simulink subsystem "Szakaszmotornelkul"  (R2024b)
settings: Solver=VariableStepAuto  StartTime=0.0  StopTime=10.0  RelTol=1e-3
undefined symbols (not defined in the file or in its folder): tau_max
settings Model: Creator=Asus  LastModifiedBy=Asus

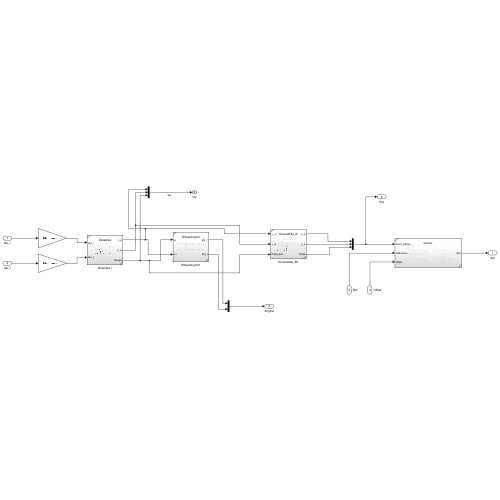
[thumbnail: Simulink's stored preview of the top-level diagram]
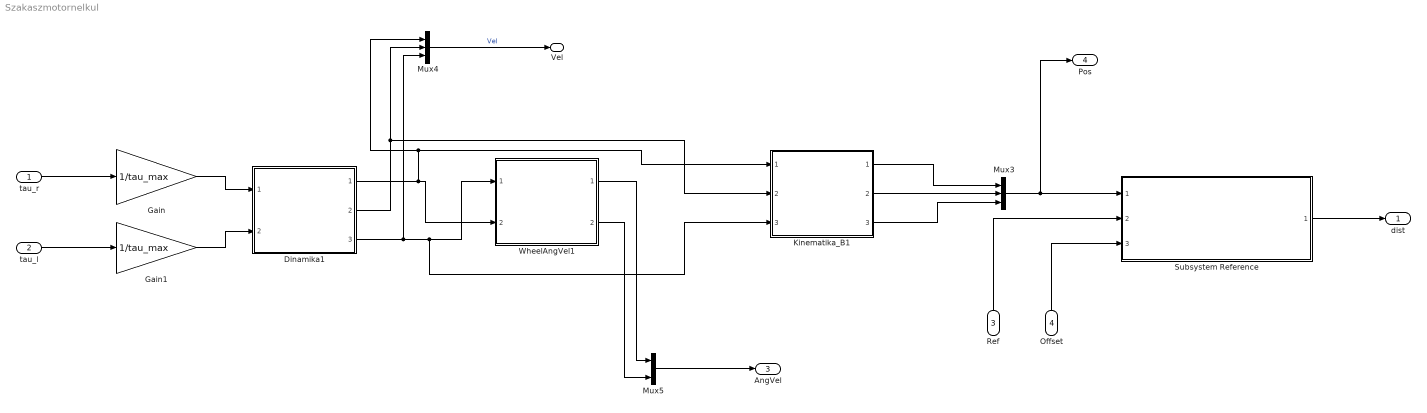
== system Szakaszmotornelkul ==
  tau_r : Inport
  tau_l : Inport  Port=2
  Ref : Inport  Port=3
  Offset : Inport  Port=4
  Dinamika1 : Subsystem  ReferencedSubsystem=Dinamika
  Gain : Gain  Gain=1/tau_max
  Gain1 : Gain  Gain=1/tau_max
  Kinematika_B1 : Subsystem  ReferencedSubsystem=Kinematika_B
  Mux3 : Mux  Inputs=3
  Mux4 : Mux  Inputs=3
  Mux5 : Mux  Inputs=2
  Subsystem Reference : Subsystem  ReferencedSubsystem=sensor
  WheelAngVel1 : Subsystem  ReferencedSubsystem=WheelAngVel
  dist : Outport
  Vel : Outport  Port=2
  AngVel : Outport  Port=3
  Pos : Outport  Port=4
  wires:
  Kinematika_B1/1 -> Mux3/1
  Dinamika1/2 -> Mux4/2, Kinematika_B1/2
  WheelAngVel1/2 -> Mux5/2
  Kinematika_B1/3 -> Mux3/3
  Dinamika1/3 -> WheelAngVel1/1, Kinematika_B1/3, Mux4/3
  Mux5/1 -> AngVel/1
  Mux4/1 -> Vel/1  "Vel"
  WheelAngVel1/1 -> Mux5/1
  Dinamika1/1 -> WheelAngVel1/2, Kinematika_B1/1, Mux4/1
  Kinematika_B1/2 -> Mux3/2
  Mux3/1 -> Pos/1, Subsystem Reference/1
  Ref/1 -> Subsystem Reference/2
  Offset/1 -> Subsystem Reference/3
  Subsystem Reference/1 -> dist/1
  tau_r/1 -> Gain/1
  tau_l/1 -> Gain1/1
  Gain/1 -> Dinamika1/1
  Gain1/1 -> Dinamika1/2
